simulink library "WECSim_Lib"  (R2019b)
settings: Solver=ode45  StartTime=0.0  StopTime=10.0  RelTol=1e-3  EnableMultiTasking=on
undefined symbols (not defined in the file): body, constraint, mooring, pto, simu, waves, X, Y, Z
libraries: nesl_utility x168, sm_lib x94, vrlib x12
(part 6 of 6)

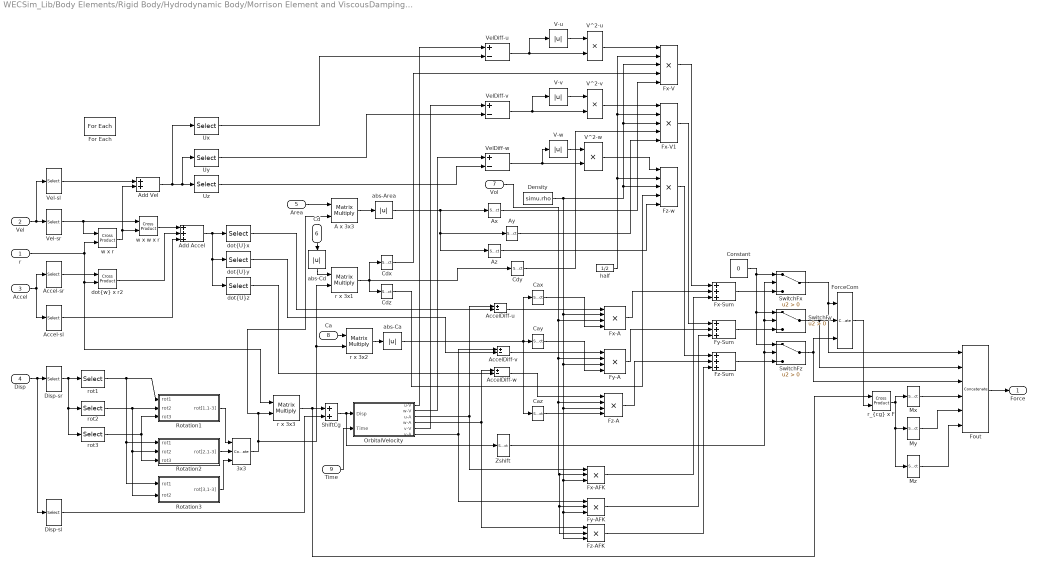
== system WECSim_Lib/Body Elements/Rigid Body/Hydrodynamic Body/Morrison Element and ViscousDampingForceCalculation/Morrison Element Variant Subsystem/Morrison Element On/Regular Wave Morison Force/MorrisonElements ==
  r : Inport  Partition=on  PartitionDimension=1  PartitionWidth=1  PartitionOffset=0
  Vel : Inport  Port=2
  Accel : Inport  Port=3
  Disp : Inport  Port=4
  Area : Inport  Port=5  Partition=on  PartitionDimension=1  PartitionWidth=1  PartitionOffset=0
  Cd : Inport  Port=6  Partition=on  PartitionDimension=1  PartitionWidth=1  PartitionOffset=0
  Vol : Inport  Port=7  Partition=on  PartitionDimension=1  PartitionWidth=1  PartitionOffset=0
  Ca : Inport  Port=8  Partition=on  PartitionDimension=1  PartitionWidth=1  PartitionOffset=0
  Time : Inport  Port=9
  3x3 : Concatenate  NumInputs=3  Mode=Multidimensional array
  A x 3x3 : Product  Multiplication=Matrix(*)
  Accel-sl : Selector  InputPortWidth=6  IndexOptions=Index vector (dialog)  Indices=[1 2 3]  OutputSizes=1
  Accel-sr : Selector  InputPortWidth=6  IndexOptions=Index vector (dialog)  Indices=[4 5 6]  OutputSizes=1
  AccelDiff-u : Sum  Inputs=+-
  AccelDiff-v : Sum  Inputs=+-
  AccelDiff-w : Sum  Inputs=+-
  Add Accel : Sum  Inputs=+++
  Add Vel : Sum
  Ax : Selector  InputPortWidth=3  IndexOptions=Index vector (dialog)  Indices=[1]  OutputSizes=1
  Ay : Selector  InputPortWidth=3  IndexOptions=Index vector (dialog)  Indices=[2]  OutputSizes=1
  Az : Selector  InputPortWidth=3  IndexOptions=Index vector (dialog)  Indices=[3]  OutputSizes=1
  Cax : Selector  InputPortWidth=3  IndexOptions=Index vector (dialog)  Indices=[1]  OutputSizes=1
  Cay : Selector  InputPortWidth=3  IndexOptions=Index vector (dialog)  Indices=[2]  OutputSizes=1
  Caz : Selector  InputPortWidth=3  IndexOptions=Index vector (dialog)  Indices=[3]  OutputSizes=1
  Cdx : Selector  InputPortWidth=3  IndexOptions=Index vector (dialog)  Indices=[1]  OutputSizes=1
  Cdy : Selector  InputPortWidth=3  IndexOptions=Index vector (dialog)  Indices=[2]  OutputSizes=1
  Cdz : Selector  InputPortWidth=3  IndexOptions=Index vector (dialog)  Indices=[3]  OutputSizes=1
  Constant : Constant  Value=0
  Density : Constant  Value=simu.rho
  Disp-sl : Selector  InputPortWidth=6  IndexOptions=Index vector (dialog)  Indices=[1 2 3]  OutputSizes=1
  Disp-sr : Selector  InputPortWidth=6  IndexOptions=Index vector (dialog)  Indices=[4 5 6]  OutputSizes=1
  For Each : ForEach  DisableCoverage=on
  ForceCom : Concatenate  NumInputs=3  ConcatenateDimension=2
  Fout : Concatenate  NumInputs=6  Mode=Multidimensional array  ConcatenateDimension=2
  Fx-A : Product  Inputs=4
  Fx-AFK : Product  Inputs=3
  Fx-Sum : Sum  Inputs=+++
  Fx-V : Product  Inputs=5
  Fx-V1 : Product  Inputs=5
  Fy-A : Product  Inputs=4
  Fy-AFK : Product  Inputs=3
  Fy-Sum : Sum  Inputs=+++
  Fz-A : Product  Inputs=4
  Fz-AFK : Product  Inputs=3
  Fz-Sum : Sum  Inputs=+++
  Fz-w : Product  Inputs=5
  Mx : Selector  InputPortWidth=3  IndexOptions=Index vector (dialog)  Indices=[1]  OutputSizes=1
  My : Selector  InputPortWidth=3  IndexOptions=Index vector (dialog)  Indices=[2]  OutputSizes=1
  Mz : Selector  InputPortWidth=3  IndexOptions=Index vector (dialog)  Indices=[3]  OutputSizes=1
  OrbitalVelocity : Subsystem
  Rotation1 : Subsystem
  Rotation2 : Subsystem
  Rotation3 : Subsystem
  ShiftCg : Sum
  SwitchFx : Switch  Criteria=u2 > Threshold
  SwitchFy : Switch  Criteria=u2 > Threshold
  SwitchFz : Switch  Criteria=u2 > Threshold
  Ux : Selector  InputPortWidth=3  IndexOptions=Index vector (dialog)  Indices=[1]  OutputSizes=1
  Uy : Selector  InputPortWidth=3  IndexOptions=Index vector (dialog)  Indices=[2]  OutputSizes=1
  Uz : Selector  InputPortWidth=3  IndexOptions=Index vector (dialog)  Indices=[3]  OutputSizes=1
  V-u : Abs
  V-v : Abs
  V-w : Abs
  V^2-u : Product
  V^2-v : Product
  V^2-w : Product
  Vel-sl : Selector  InputPortWidth=6  IndexOptions=Index vector (dialog)  Indices=[1 2 3]  OutputSizes=1
  "Vel-sr " : Selector  InputPortWidth=6  IndexOptions=Index vector (dialog)  Indices=[4 5 6]  OutputSizes=1
  VelDiff-u : Sum  Inputs=+-
  VelDiff-v : Sum  Inputs=+-
  VelDiff-w : Sum  Inputs=+-
  Zshift : Selector  InputPortWidth=3  IndexOptions=Index vector (dialog)  Indices=[3]  OutputSizes=1
  abs-Area : Abs
  abs-Ca : Abs
  abs-Cd : Abs
  "dot{U}x" : Selector  InputPortWidth=3  IndexOptions=Index vector (dialog)  Indices=[1]  OutputSizes=1
  "dot{U}y" : Selector  InputPortWidth=3  IndexOptions=Index vector (dialog)  Indices=[2]  OutputSizes=1
  "dot{U}z" : Selector  InputPortWidth=3  IndexOptions=Index vector (dialog)  Indices=[3]  OutputSizes=1
  "dot{w} x r2" : vrlib/Utilities/Cross Product
      settings: SourceProductName=Simulink
  half : Constant  Value=1/2
  r x 3x1 : Product  Multiplication=Matrix(*)
  r x 3x2 : Product  Multiplication=Matrix(*)
  r x 3x3 : Product  Multiplication=Matrix(*)
  "r_{cg} x F" : vrlib/Utilities/Cross Product
      settings: SourceProductName=Simulink
  rot1 : Selector  InputPortWidth=3  IndexOptions=Index vector (dialog)  Indices=[1]  OutputSizes=1
  rot2 : Selector  InputPortWidth=3  IndexOptions=Index vector (dialog)  Indices=[2]  OutputSizes=1
  rot3 : Selector  InputPortWidth=3  IndexOptions=Index vector (dialog)  Indices=[3]  OutputSizes=1
  w x r : vrlib/Utilities/Cross Product
      settings: SourceProductName=Simulink
  w x w x r : vrlib/Utilities/Cross Product
      settings: SourceProductName=Simulink
  Force : Outport  PortDimensions=[1 6]  ConcatenationDimension=1
  wires:
  Vel/1 -> Vel-sl/1, "Vel-sr "/1
  w x r/1 -> Add Vel/2, w x w x r/2
  w x w x r/1 -> Add Accel/1
  "Vel-sr "/1 -> w x w x r/1, w x r/1
  r/1 -> r x 3x3/1, "dot{w} x r2"/2, w x r/2
  Accel/1 -> Accel-sl/1, Accel-sr/1
  Accel-sr/1 -> "dot{w} x r2"/1
  "dot{w} x r2"/1 -> Add Accel/2
  Accel-sl/1 -> Add Accel/3
  Add Accel/1 -> "dot{U}z"/1, "dot{U}y"/1, "dot{U}x"/1
  Vel-sl/1 -> Add Vel/1
  Disp/1 -> Disp-sl/1, Disp-sr/1
  Disp-sr/1 -> rot3/1, rot2/1, rot1/1
  rot3/1 -> Rotation2/3(rot3), Rotation1/3(rot3)
  rot1/1 -> Rotation3/1(rot1), Rotation2/1(rot1), Rotation1/1(rot1)
  rot2/1 -> Rotation3/2(rot2), Rotation2/2(rot2), Rotation1/2(rot2)
  Rotation2/1(rot[2,1-3]) -> 3x3/2
  Rotation1/1(rot[1,1-3]) -> 3x3/1
  Rotation3/1(rot[3,1-3]) -> 3x3/3
  r x 3x3/1 -> "r_{cg} x F"/1, ShiftCg/1
  Disp-sl/1 -> ShiftCg/2
  ShiftCg/1 -> Zshift/1, OrbitalVelocity/1(Disp)
  "dot{U}y"/1 -> AccelDiff-v/2
  "dot{U}x"/1 -> AccelDiff-u/2
  OrbitalVelocity/3(u-A) -> AccelDiff-u/1, Fx-AFK/1
  "dot{U}z"/1 -> AccelDiff-w/2
  Add Vel/1 -> Uy/1, Uz/1, Ux/1
  Uy/1 -> VelDiff-v/2
  Ux/1 -> VelDiff-u/2
  Uz/1 -> VelDiff-w/2
  OrbitalVelocity/1(u-V) -> VelDiff-u/1
  OrbitalVelocity/2(w-V) -> VelDiff-w/1
  VelDiff-w/1 -> V-w/1, V^2-w/2
  V^2-u/1 -> Fx-V/1
  half/1 -> Fz-w/2, Fx-V1/2, Fx-V/2
  Density/1 -> Fy-A/3, Fy-AFK/3, Fz-AFK/3, Fx-AFK/3, Fz-A/3, Fx-A/2, Fz-w/3, Fx-V1/3, Fx-V/3
  V^2-w/1 -> Fz-w/1
  AccelDiff-u/1 -> Fx-A/1
  Vol/1 -> Fy-A/2, Fy-AFK/2, Fz-AFK/2, Fx-AFK/2, Fz-A/2, Fx-A/3
  AccelDiff-w/1 -> Fz-A/1
  OrbitalVelocity/4(w-A) -> Fz-AFK/1, AccelDiff-w/1
  Fx-V/1 -> Fx-Sum/1
  Fx-A/1 -> Fx-Sum/2
  Fx-AFK/1 -> Fx-Sum/3
  Fz-w/1 -> Fz-Sum/1
  Fz-A/1 -> Fz-Sum/2
  Fz-AFK/1 -> Fz-Sum/3
  "r_{cg} x F"/1 -> Mz/1, My/1, Mx/1
  Mx/1 -> Fout/4
  My/1 -> Fout/5
  Mz/1 -> Fout/6
  3x3/1 -> A x 3x3/2, r x 3x3/2, r x 3x2/2, r x 3x1/2
  V-u/1 -> V^2-u/1
  VelDiff-u/1 -> V-u/1, V^2-u/2
  Zshift/1 -> SwitchFy/2, SwitchFx/2, SwitchFz/2
  SwitchFz/1 -> ForceCom/3, Fout/3
  SwitchFx/1 -> Fout/1, ForceCom/1
  Fx-Sum/1 -> SwitchFx/3
  Fz-Sum/1 -> SwitchFz/3
  Az/1 -> Fz-w/5
  Area/1 -> A x 3x3/1
  Ax/1 -> Fx-V/5
  Cdx/1 -> Fx-V/4
  Cdz/1 -> Fz-w/4
  A x 3x3/1 -> abs-Area/1
  abs-Area/1 -> Ay/1, Az/1, Ax/1
  ForceCom/1 -> "r_{cg} x F"/2
  Fout/1 -> Force/1
  Caz/1 -> Fz-A/4
  Cax/1 -> Fx-A/4
  Cd/1 -> abs-Cd/1
  r x 3x1/1 -> Cdy/1, Cdz/1, Cdx/1
  Ca/1 -> r x 3x2/1
  r x 3x2/1 -> abs-Ca/1
  OrbitalVelocity/6(v-A) -> AccelDiff-v/1, Fy-AFK/1
  V^2-v/1 -> Fx-V1/1
  V-v/1 -> V^2-v/1
  VelDiff-v/1 -> V-v/1, V^2-v/2
  OrbitalVelocity/5(v-V) -> VelDiff-v/1
  Ay/1 -> Fx-V1/5
  Cdy/1 -> Fx-V1/4
  SwitchFy/1 -> Fout/2, ForceCom/2
  Fy-Sum/1 -> SwitchFy/3
  Fy-AFK/1 -> Fy-Sum/3
  AccelDiff-v/1 -> Fy-A/1
  Cay/1 -> Fy-A/4
  Fy-A/1 -> Fy-Sum/2
  Fx-V1/1 -> Fy-Sum/1
  Constant/1 -> SwitchFy/1, SwitchFz/1, SwitchFx/1
  V-w/1 -> V^2-w/1
  abs-Ca/1 -> Cax/1, Cay/1, Caz/1
  abs-Cd/1 -> r x 3x1/1
  Time/1 -> OrbitalVelocity/2(Time)

== system WECSim_Lib/Body Elements/Rigid Body/Hydrodynamic Body/Morrison Element and ViscousDampingForceCalculation/Morrison Element Variant Subsystem/Morrison Element On/Irregular Wave Morison Force/MorrisonElements/MorisonElementIrregular ==
  Disp : Inport
  waves.kirr : Inport  Port=2  Partition=on  PartitionDimension=1  PartitionWidth=1  PartitionOffset=0
  waves.w : Inport  Port=3  Partition=on  PartitionDimension=1  PartitionWidth=1  PartitionOffset=0
  waves.A : Inport  Port=4  Partition=on  PartitionDimension=1  PartitionWidth=1  PartitionOffset=0
  waves.Phase : Inport  Port=5  Partition=on  PartitionDimension=1  PartitionWidth=1  PartitionOffset=0
  Time : Inport  Port=6
  For Each : ForEach  DisableCoverage=on
  MATLAB Function : MATLAB Function  TreatAsAtomicUnit=on
  gravity : Constant  Value=simu.g  VectorParams1D=off
  rampTime : Constant  Value=simu.rampTime  VectorParams1D=off
  waterDepth : Constant  Value=waves.waterDepth  VectorParams1D=off
  waveDirection : Constant  Value=waves.waveDir  VectorParams1D=off
  u-V : Outport  ConcatenationDimension=1
  w-V : Outport  Port=2  ConcatenationDimension=1
  x-A : Outport  Port=3  ConcatenationDimension=1
  w-A : Outport  Port=4  ConcatenationDimension=1
  v-V : Outport  Port=5  ConcatenationDimension=1
  y-A : Outport  Port=6  ConcatenationDimension=1
  wires:
  gravity/1 -> MATLAB Function/10(g)
  waterDepth/1 -> MATLAB Function/9(waterDepth)
  waveDirection/1 -> MATLAB Function/8(waveDir)
  rampTime/1 -> MATLAB Function/7(rampT)
  Disp/1 -> MATLAB Function/1(disp)
  waves.w/1 -> MATLAB Function/3(waveFreq)
  waves.A/1 -> MATLAB Function/4(waveAmp)
  waves.Phase/1 -> MATLAB Function/5(phase)
  MATLAB Function/1(u) -> u-V/1
  waves.kirr/1 -> MATLAB Function/2(waveNumber)
  Time/1 -> MATLAB Function/6(time)
  MATLAB Function/2(v) -> v-V/1
  MATLAB Function/5(ya) -> y-A/1
  MATLAB Function/6(za) -> w-A/1
  MATLAB Function/4(xa) -> x-A/1
  MATLAB Function/3(w) -> w-V/1

== system WECSim_Lib/Body Elements/Rigid Body/Hydrodynamic Body/Morrison Element and ViscousDampingForceCalculation/Morrison Element Variant Subsystem/Morrison Element On/Irregular Wave Morison Force/MorrisonElements/Rotation1 ==
  rot1 : Inport
  rot2 : Inport  Port=2
  rot3 : Inport  Port=3
  2 : Product
  3 : Product  Inputs=3
  7 : Product
  8 : Product  Inputs=3
  Combine : Concatenate  NumInputs=3  Mode=Multidimensional array  ConcatenateDimension=2
  Trigonometric Function{,1..2,6,9,11} (6 alike) : Trigonometry  Operator=cos
  Trigonometric Function{3..5,7..8,10} (6 alike) : Trigonometry
  rot11 : Product
  rot12 : Sum
  rot13 : Sum  Inputs=+-
  rot[1,1-3] : Outport
  wires:
  Trigonometric Function/1 -> rot11/1
  Trigonometric Function1/1 -> rot11/2
  rot11/1 -> Combine/1
  Trigonometric Function2/1 -> 2/1
  Trigonometric Function3/1 -> 2/2
  Trigonometric Function4/1 -> 3/1
  Trigonometric Function5/1 -> 3/2
  Trigonometric Function6/1 -> 3/3
  2/1 -> rot12/1
  3/1 -> rot12/2
  rot12/1 -> Combine/2
  Combine/1 -> rot[1,1-3]/1
  rot2/1 -> Trigonometric Function/1, Trigonometric Function5/1, Trigonometric Function10/1
  rot3/1 -> Trigonometric Function1/1, Trigonometric Function3/1, Trigonometric Function6/1, Trigonometric Function11/1, Trigonometric Function8/1
  rot1/1 -> Trigonometric Function2/1, Trigonometric Function4/1, Trigonometric Function9/1, Trigonometric Function7/1
  Trigonometric Function7/1 -> 7/1
  Trigonometric Function8/1 -> 7/2
  Trigonometric Function9/1 -> 8/1
  Trigonometric Function10/1 -> 8/2
  Trigonometric Function11/1 -> 8/3
  7/1 -> rot13/1
  8/1 -> rot13/2
  rot13/1 -> Combine/3

== system WECSim_Lib/Body Elements/Rigid Body/Hydrodynamic Body/Morrison Element and ViscousDampingForceCalculation/Morrison Element Variant Subsystem/Morrison Element On/Irregular Wave Morison Force/MorrisonElements/Rotation2 ==
  rot1 : Inport
  rot2 : Inport  Port=2
  rot3 : Inport  Port=3
  2 : Product
  3 : Product  Inputs=3
  7 : Product
  8 : Product  Inputs=3
  Combine : Concatenate  NumInputs=3  Mode=Multidimensional array  ConcatenateDimension=2
  Gain : Gain  Gain=-1
  Trigonometric Function{,2..3,8..9} (5 alike) : Trigonometry  Operator=cos
  Trigonometric Function{1,4..7,10..11} (7 alike) : Trigonometry
  rot11 : Product
  rot12 : Sum  Inputs=+-
  rot13 : Sum
  rot[2,1-3] : Outport
  wires:
  Trigonometric Function/1 -> Gain/1
  Trigonometric Function1/1 -> rot11/2
  rot11/1 -> Combine/1
  Trigonometric Function2/1 -> 2/1
  Trigonometric Function3/1 -> 2/2
  Trigonometric Function4/1 -> 3/1
  Trigonometric Function5/1 -> 3/2
  Trigonometric Function6/1 -> 3/3
  2/1 -> rot12/1
  3/1 -> rot12/2
  rot12/1 -> Combine/2
  Combine/1 -> rot[2,1-3]/1
  rot2/1 -> Trigonometric Function/1, Trigonometric Function5/1, Trigonometric Function10/1
  rot3/1 -> Trigonometric Function1/1, Trigonometric Function3/1, Trigonometric Function6/1, Trigonometric Function11/1, Trigonometric Function8/1
  rot1/1 -> Trigonometric Function2/1, Trigonometric Function4/1, Trigonometric Function9/1, Trigonometric Function7/1
  Trigonometric Function7/1 -> 7/1
  Trigonometric Function8/1 -> 7/2
  Trigonometric Function9/1 -> 8/1
  Trigonometric Function10/1 -> 8/2
  Trigonometric Function11/1 -> 8/3
  7/1 -> rot13/1
  8/1 -> rot13/2
  rot13/1 -> Combine/3
  Gain/1 -> rot11/1

== system WECSim_Lib/Body Elements/Rigid Body/Hydrodynamic Body/Morrison Element and ViscousDampingForceCalculation/Morrison Element Variant Subsystem/Morrison Element On/Irregular Wave Morison Force/MorrisonElements/Rotation3 ==
  rot1 : Inport
  rot2 : Inport  Port=2
  2 : Product
  7 : Product
  Combine : Concatenate  NumInputs=3  Mode=Multidimensional array  ConcatenateDimension=2
  Gain1 : Gain  Gain=-1
  TrigFun1 : Trigonometry
  TrigFun2 : Trigonometry
  TrigFun3 : Trigonometry  Operator=cos
  TrigFun4 : Trigonometry  Operator=cos
  TrigFun5 : Trigonometry  Operator=cos
  rot[3,1-3] : Outport
  wires:
  TrigFun1/1 -> Combine/1
  TrigFun3/1 -> 2/2
  2/1 -> Combine/2
  Combine/1 -> rot[3,1-3]/1
  rot2/1 -> TrigFun5/1, TrigFun3/1, TrigFun1/1
  TrigFun4/1 -> 7/1
  TrigFun5/1 -> 7/2
  rot1/1 -> TrigFun2/1, TrigFun4/1
  7/1 -> Combine/3
  TrigFun2/1 -> Gain1/1
  Gain1/1 -> 2/1

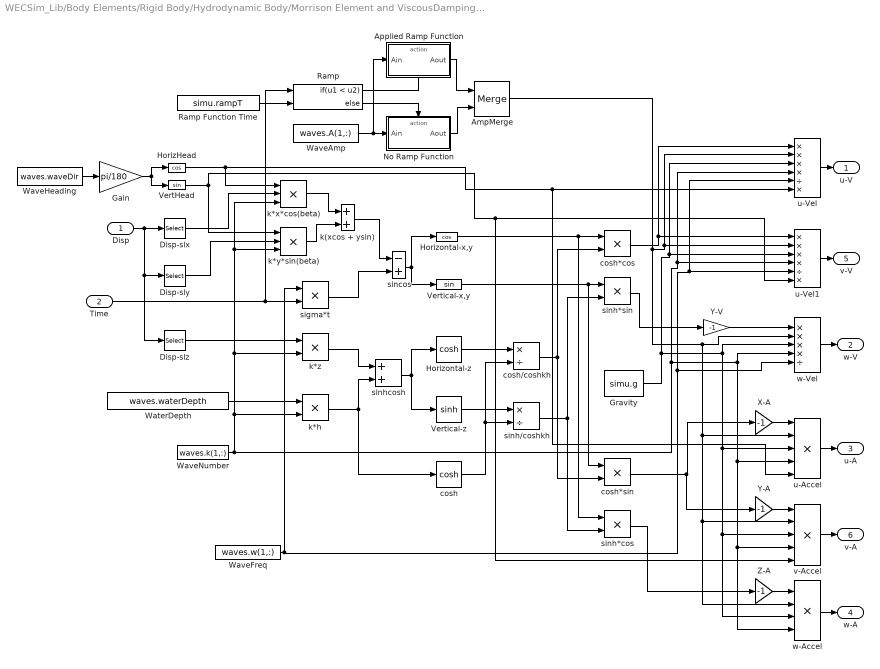
== system WECSim_Lib/Body Elements/Rigid Body/Hydrodynamic Body/Morrison Element and ViscousDampingForceCalculation/Morrison Element Variant Subsystem/Morrison Element On/No Wave Morison Force/MorrisonElements/OrbitalVelocity ==
  Disp : Inport
  Time : Inport  Port=2
  AmpMerge : Merge
  Applied Ramp Function : Subsystem  TreatAsAtomicUnit=on
  Disp-slx : Selector  InputPortWidth=3  IndexOptions=Index vector (dialog)  Indices=[1]  OutputSizes=1
  Disp-sly : Selector  InputPortWidth=3  IndexOptions=Index vector (dialog)  Indices=[2]  OutputSizes=1
  Disp-slz : Selector  InputPortWidth=3  IndexOptions=Index vector (dialog)  Indices=[3]  OutputSizes=1
  Gain : Gain  Gain=pi/180
  Gravity : Constant  Value=simu.g
  HorizHead : Trigonometry  Operator=cos
  Horizontal-x,y : Trigonometry  Operator=cos
  Horizontal-z : Trigonometry  Operator=cosh
  No Ramp Function : Subsystem  TreatAsAtomicUnit=on
  Ramp : If  NumInputs=2  IfExpression=u1 < u2
  Ramp Function Time : Constant  Value=simu.rampT
  VertHead : Trigonometry
  Vertical-x,y : Trigonometry
  Vertical-z : Trigonometry  Operator=sinh
  WaterDepth : Constant  Value=waves.waterDepth
  WaveAmp : Constant  Value=waves.A(1,:)
  WaveFreq : Constant  Value=waves.w(1,:)
  WaveHeading : Constant  Value=waves.waveDir
  WaveNumber : Constant  Value=waves.k(1,:)
  X-A : Gain  Gain=-1
  Y-A : Gain  Gain=-1
  Y-V : Gain  Gain=-1
  Z-A : Gain  Gain=-1
  cosh : Trigonometry  Operator=cosh
  cosh*cos : Product  Inputs=**
  cosh*sin : Product  Inputs=**
  cosh/coshkh : Product  Inputs=*/
  k(xcos + ysin) : Sum
  k*h : Product
  k*x*cos(beta) : Product  Inputs=3
  k*y*sin(beta) : Product  Inputs=3
  k*z : Product
  sigma*t : Product
  sincos : Sum  Inputs=-+
  sinh*cos : Product  Inputs=**
  sinh*sin : Product  Inputs=**
  sinh/coshkh : Product  Inputs=*/
  sinhcosh : Sum
  u-Accel : Product  Inputs=*****
  u-Vel : Product  Inputs=****/*
  u-Vel1 : Product  Inputs=****/*
  v-Accel : Product  Inputs=*****
  w-Accel : Product  Inputs=****
  w-Vel : Product  Inputs=****/
  u-V : Outport
  w-V : Outport  Port=2
  u-A : Outport  Port=3
  w-A : Outport  Port=4
  v-V : Outport  Port=5
  v-A : Outport  Port=6
  wires:
  Disp/1 -> Disp-slz/1, Disp-sly/1, Disp-slx/1
  WaveNumber/1 -> k*h/2, k*z/2, k*y*sin(beta)/3, k*x*cos(beta)/3, w-Vel/4, v-Accel/4, w-Accel/4, u-Accel/4, u-Vel1/4, u-Vel/4
  WaterDepth/1 -> k*h/1
  sigma*t/1 -> sincos/2
  sincos/1 -> Vertical-x,y/1, Horizontal-x,y/1
  k*z/1 -> sinhcosh/1
  k*h/1 -> cosh/1, sinhcosh/2
  sinhcosh/1 -> Vertical-z/1, Horizontal-z/1
  Horizontal-z/1 -> cosh/coshkh/1
  cosh/1 -> sinh/coshkh/2, cosh/coshkh/2
  Vertical-z/1 -> sinh/coshkh/1
  Vertical-x,y/1 -> cosh*sin/1, sinh*sin/1
  sinh/coshkh/1 -> sinh*cos/2, sinh*sin/2
  Horizontal-x,y/1 -> sinh*cos/1, cosh*cos/1
  cosh/coshkh/1 -> cosh*cos/2, cosh*sin/2
  Disp-sly/1 -> k*y*sin(beta)/2
  cosh*cos/1 -> u-Vel1/1, u-Vel/1
  AmpMerge/1 -> w-Vel/2, w-Accel/2, v-Accel/2, u-Accel/2, u-Vel1/2, u-Vel/2
  Gravity/1 -> w-Vel/3, v-Accel/3, w-Accel/3, u-Accel/3, u-Vel1/3, u-Vel/3
  sinh*sin/1 -> Y-V/1
  Y-V/1 -> w-Vel/1
  X-A/1 -> u-Accel/1
  Z-A/1 -> w-Accel/1
  w-Vel/1 -> w-V/1
  u-Accel/1 -> u-A/1
  w-Accel/1 -> w-A/1
  cosh*sin/1 -> Y-A/1, X-A/1
  sinh*cos/1 -> Z-A/1
  Ramp Function Time/1 -> Ramp/2
  Ramp/2 -> No Ramp Function/Action
  Ramp/1 -> Applied Ramp Function/Action
  Time/1 -> Ramp/1, sigma*t/2
  No Ramp Function/1(Aout) -> AmpMerge/2
  Applied Ramp Function/1(Aout) -> AmpMerge/1
  Disp-slz/1 -> k*z/1
  WaveFreq/1 -> w-Vel/5, u-Vel1/5, u-Vel/5, sigma*t/1
  WaveAmp/1 -> Applied Ramp Function/1(Ain), No Ramp Function/1(Ain)
  WaveHeading/1 -> Gain/1
  Gain/1 -> HorizHead/1, VertHead/1
  Disp-slx/1 -> k*x*cos(beta)/2
  HorizHead/1 -> u-Accel/5, u-Vel/6, k*x*cos(beta)/1
  VertHead/1 -> k*y*sin(beta)/1, u-Vel1/6, v-Accel/5
  k*y*sin(beta)/1 -> k(xcos + ysin)/2
  k*x*cos(beta)/1 -> k(xcos + ysin)/1
  k(xcos + ysin)/1 -> sincos/1
  u-Vel1/1 -> v-V/1
  u-Vel/1 -> u-V/1
  Y-A/1 -> v-Accel/1
  v-Accel/1 -> v-A/1

== system WECSim_Lib/Body Elements/Rigid Body/Hydrodynamic Body/Morrison Element and ViscousDampingForceCalculation/Morrison Element Variant Subsystem/Morrison Element On/No Wave Morison Force/MorrisonElements/Rotation1 ==
  rot1 : Inport
  rot2 : Inport  Port=2
  rot3 : Inport  Port=3
  2 : Product
  3 : Product  Inputs=3
  7 : Product
  8 : Product  Inputs=3
  Combine : Concatenate  NumInputs=3  Mode=Multidimensional array  ConcatenateDimension=2
  Trigonometric Function{,1..2,6,9,11} (6 alike) : Trigonometry  Operator=cos
  Trigonometric Function{3..5,7..8,10} (6 alike) : Trigonometry
  rot11 : Product
  rot12 : Sum
  rot13 : Sum  Inputs=+-
  rot[1,1-3] : Outport
  wires:
  Trigonometric Function/1 -> rot11/1
  Trigonometric Function1/1 -> rot11/2
  rot11/1 -> Combine/1
  Trigonometric Function2/1 -> 2/1
  Trigonometric Function3/1 -> 2/2
  Trigonometric Function4/1 -> 3/1
  Trigonometric Function5/1 -> 3/2
  Trigonometric Function6/1 -> 3/3
  2/1 -> rot12/1
  3/1 -> rot12/2
  rot12/1 -> Combine/2
  Combine/1 -> rot[1,1-3]/1
  rot2/1 -> Trigonometric Function/1, Trigonometric Function5/1, Trigonometric Function10/1
  rot3/1 -> Trigonometric Function1/1, Trigonometric Function3/1, Trigonometric Function6/1, Trigonometric Function11/1, Trigonometric Function8/1
  rot1/1 -> Trigonometric Function2/1, Trigonometric Function4/1, Trigonometric Function9/1, Trigonometric Function7/1
  Trigonometric Function7/1 -> 7/1
  Trigonometric Function8/1 -> 7/2
  Trigonometric Function9/1 -> 8/1
  Trigonometric Function10/1 -> 8/2
  Trigonometric Function11/1 -> 8/3
  7/1 -> rot13/1
  8/1 -> rot13/2
  rot13/1 -> Combine/3

== system WECSim_Lib/Body Elements/Rigid Body/Hydrodynamic Body/Morrison Element and ViscousDampingForceCalculation/Morrison Element Variant Subsystem/Morrison Element On/No Wave Morison Force/MorrisonElements/Rotation2 ==
  rot1 : Inport
  rot2 : Inport  Port=2
  rot3 : Inport  Port=3
  2 : Product
  3 : Product  Inputs=3
  7 : Product
  8 : Product  Inputs=3
  Combine : Concatenate  NumInputs=3  Mode=Multidimensional array  ConcatenateDimension=2
  Gain : Gain  Gain=-1
  Trigonometric Function{,2..3,8..9} (5 alike) : Trigonometry  Operator=cos
  Trigonometric Function{1,4..7,10..11} (7 alike) : Trigonometry
  rot11 : Product
  rot12 : Sum  Inputs=+-
  rot13 : Sum
  rot[2,1-3] : Outport
  wires:
  Trigonometric Function/1 -> Gain/1
  Trigonometric Function1/1 -> rot11/2
  rot11/1 -> Combine/1
  Trigonometric Function2/1 -> 2/1
  Trigonometric Function3/1 -> 2/2
  Trigonometric Function4/1 -> 3/1
  Trigonometric Function5/1 -> 3/2
  Trigonometric Function6/1 -> 3/3
  2/1 -> rot12/1
  3/1 -> rot12/2
  rot12/1 -> Combine/2
  Combine/1 -> rot[2,1-3]/1
  rot2/1 -> Trigonometric Function/1, Trigonometric Function5/1, Trigonometric Function10/1
  rot3/1 -> Trigonometric Function1/1, Trigonometric Function3/1, Trigonometric Function6/1, Trigonometric Function11/1, Trigonometric Function8/1
  rot1/1 -> Trigonometric Function2/1, Trigonometric Function4/1, Trigonometric Function9/1, Trigonometric Function7/1
  Trigonometric Function7/1 -> 7/1
  Trigonometric Function8/1 -> 7/2
  Trigonometric Function9/1 -> 8/1
  Trigonometric Function10/1 -> 8/2
  Trigonometric Function11/1 -> 8/3
  7/1 -> rot13/1
  8/1 -> rot13/2
  rot13/1 -> Combine/3
  Gain/1 -> rot11/1

== system WECSim_Lib/Body Elements/Rigid Body/Hydrodynamic Body/Morrison Element and ViscousDampingForceCalculation/Morrison Element Variant Subsystem/Morrison Element On/No Wave Morison Force/MorrisonElements/Rotation3 ==
  rot1 : Inport
  rot2 : Inport  Port=2
  2 : Product
  7 : Product
  Combine : Concatenate  NumInputs=3  Mode=Multidimensional array  ConcatenateDimension=2
  Gain1 : Gain  Gain=-1
  TrigFun1 : Trigonometry
  TrigFun2 : Trigonometry
  TrigFun3 : Trigonometry  Operator=cos
  TrigFun4 : Trigonometry  Operator=cos
  TrigFun5 : Trigonometry  Operator=cos
  rot[3,1-3] : Outport
  wires:
  TrigFun1/1 -> Combine/1
  TrigFun3/1 -> 2/2
  2/1 -> Combine/2
  Combine/1 -> rot[3,1-3]/1
  rot2/1 -> TrigFun5/1, TrigFun3/1, TrigFun1/1
  TrigFun4/1 -> 7/1
  TrigFun5/1 -> 7/2
  rot1/1 -> TrigFun2/1, TrigFun4/1
  7/1 -> Combine/3
  TrigFun2/1 -> Gain1/1
  Gain1/1 -> 2/1

== system WECSim_Lib/Body Elements/Rigid Body/Hydrodynamic Body/Morrison Element and ViscousDampingForceCalculation/Morrison Element Variant Subsystem/Morrison Element On/Regular Wave Morison Force/MorrisonElements/OrbitalVelocity ==
  Disp : Inport
  Time : Inport  Port=2
  MATLAB Function : MATLAB Function  TreatAsAtomicUnit=on
  WaveAmp : Constant  Value=waves.A(1,:)
  WaveFreq : Constant  Value=waves.w(1,:)
  WaveNumber : Constant  Value=waves.k(1,:)
  gravity : Constant  Value=simu.g  VectorParams1D=off
  phase : Constant  Value=0
  rampTime : Constant  Value=simu.rampTime  VectorParams1D=off
  waterDepth : Constant  Value=waves.waterDepth  VectorParams1D=off
  waveDirection : Constant  Value=waves.waveDir  VectorParams1D=off
  u-V : Outport
  w-V : Outport  Port=2
  u-A : Outport  Port=3
  w-A : Outport  Port=4
  v-V : Outport  Port=5
  v-A : Outport  Port=6
  wires:
  Disp/1 -> MATLAB Function/1(disp)
  phase/1 -> MATLAB Function/5(randPhase)
  WaveNumber/1 -> MATLAB Function/2(waveNumber)
  WaveFreq/1 -> MATLAB Function/3(waveFreq)
  WaveAmp/1 -> MATLAB Function/4(waveAmp)
  Time/1 -> MATLAB Function/6(time)
  gravity/1 -> MATLAB Function/10(g)
  waterDepth/1 -> MATLAB Function/9(waterDepth)
  waveDirection/1 -> MATLAB Function/8(waveDir)
  rampTime/1 -> MATLAB Function/7(rampT)
  MATLAB Function/3(w) -> w-V/1
  MATLAB Function/4(xa) -> u-A/1
  MATLAB Function/6(za) -> w-A/1
  MATLAB Function/2(v) -> v-V/1
  MATLAB Function/1(u) -> u-V/1
  MATLAB Function/5(ya) -> v-A/1

== system WECSim_Lib/Body Elements/Rigid Body/Hydrodynamic Body/Morrison Element and ViscousDampingForceCalculation/Morrison Element Variant Subsystem/Morrison Element On/Regular Wave Morison Force/MorrisonElements/Rotation1 ==
  rot1 : Inport
  rot2 : Inport  Port=2
  rot3 : Inport  Port=3
  2 : Product
  3 : Product  Inputs=3
  7 : Product
  8 : Product  Inputs=3
  Combine : Concatenate  NumInputs=3  Mode=Multidimensional array  ConcatenateDimension=2
  Trigonometric Function{,1..2,6,9,11} (6 alike) : Trigonometry  Operator=cos
  Trigonometric Function{3..5,7..8,10} (6 alike) : Trigonometry
  rot11 : Product
  rot12 : Sum
  rot13 : Sum  Inputs=+-
  rot[1,1-3] : Outport
  wires:
  Trigonometric Function/1 -> rot11/1
  Trigonometric Function1/1 -> rot11/2
  rot11/1 -> Combine/1
  Trigonometric Function2/1 -> 2/1
  Trigonometric Function3/1 -> 2/2
  Trigonometric Function4/1 -> 3/1
  Trigonometric Function5/1 -> 3/2
  Trigonometric Function6/1 -> 3/3
  2/1 -> rot12/1
  3/1 -> rot12/2
  rot12/1 -> Combine/2
  Combine/1 -> rot[1,1-3]/1
  rot2/1 -> Trigonometric Function/1, Trigonometric Function5/1, Trigonometric Function10/1
  rot3/1 -> Trigonometric Function1/1, Trigonometric Function3/1, Trigonometric Function6/1, Trigonometric Function11/1, Trigonometric Function8/1
  rot1/1 -> Trigonometric Function2/1, Trigonometric Function4/1, Trigonometric Function9/1, Trigonometric Function7/1
  Trigonometric Function7/1 -> 7/1
  Trigonometric Function8/1 -> 7/2
  Trigonometric Function9/1 -> 8/1
  Trigonometric Function10/1 -> 8/2
  Trigonometric Function11/1 -> 8/3
  7/1 -> rot13/1
  8/1 -> rot13/2
  rot13/1 -> Combine/3

== system WECSim_Lib/Body Elements/Rigid Body/Hydrodynamic Body/Morrison Element and ViscousDampingForceCalculation/Morrison Element Variant Subsystem/Morrison Element On/Regular Wave Morison Force/MorrisonElements/Rotation2 ==
  rot1 : Inport
  rot2 : Inport  Port=2
  rot3 : Inport  Port=3
  2 : Product
  3 : Product  Inputs=3
  7 : Product
  8 : Product  Inputs=3
  Combine : Concatenate  NumInputs=3  Mode=Multidimensional array  ConcatenateDimension=2
  Gain : Gain  Gain=-1
  Trigonometric Function{,2..3,8..9} (5 alike) : Trigonometry  Operator=cos
  Trigonometric Function{1,4..7,10..11} (7 alike) : Trigonometry
  rot11 : Product
  rot12 : Sum  Inputs=+-
  rot13 : Sum
  rot[2,1-3] : Outport
  wires:
  Trigonometric Function/1 -> Gain/1
  Trigonometric Function1/1 -> rot11/2
  rot11/1 -> Combine/1
  Trigonometric Function2/1 -> 2/1
  Trigonometric Function3/1 -> 2/2
  Trigonometric Function4/1 -> 3/1
  Trigonometric Function5/1 -> 3/2
  Trigonometric Function6/1 -> 3/3
  2/1 -> rot12/1
  3/1 -> rot12/2
  rot12/1 -> Combine/2
  Combine/1 -> rot[2,1-3]/1
  rot2/1 -> Trigonometric Function/1, Trigonometric Function5/1, Trigonometric Function10/1
  rot3/1 -> Trigonometric Function1/1, Trigonometric Function3/1, Trigonometric Function6/1, Trigonometric Function11/1, Trigonometric Function8/1
  rot1/1 -> Trigonometric Function2/1, Trigonometric Function4/1, Trigonometric Function9/1, Trigonometric Function7/1
  Trigonometric Function7/1 -> 7/1
  Trigonometric Function8/1 -> 7/2
  Trigonometric Function9/1 -> 8/1
  Trigonometric Function10/1 -> 8/2
  Trigonometric Function11/1 -> 8/3
  7/1 -> rot13/1
  8/1 -> rot13/2
  rot13/1 -> Combine/3
  Gain/1 -> rot11/1

== system WECSim_Lib/Body Elements/Rigid Body/Hydrodynamic Body/Morrison Element and ViscousDampingForceCalculation/Morrison Element Variant Subsystem/Morrison Element On/Regular Wave Morison Force/MorrisonElements/Rotation3 ==
  rot1 : Inport
  rot2 : Inport  Port=2
  2 : Product
  7 : Product
  Combine : Concatenate  NumInputs=3  Mode=Multidimensional array  ConcatenateDimension=2
  Gain1 : Gain  Gain=-1
  TrigFun1 : Trigonometry
  TrigFun2 : Trigonometry
  TrigFun3 : Trigonometry  Operator=cos
  TrigFun4 : Trigonometry  Operator=cos
  TrigFun5 : Trigonometry  Operator=cos
  rot[3,1-3] : Outport
  wires:
  TrigFun1/1 -> Combine/1
  TrigFun3/1 -> 2/2
  2/1 -> Combine/2
  Combine/1 -> rot[3,1-3]/1
  rot2/1 -> TrigFun5/1, TrigFun3/1, TrigFun1/1
  TrigFun4/1 -> 7/1
  TrigFun5/1 -> 7/2
  rot1/1 -> TrigFun2/1, TrigFun4/1
  7/1 -> Combine/3
  TrigFun2/1 -> Gain1/1
  Gain1/1 -> 2/1

== system WECSim_Lib/Body Elements/Rigid Body/Hydrodynamic Body/Morrison Element and ViscousDampingForceCalculation/Morrison Element Variant Subsystem/Morrison Element On/No Wave Morison Force/MorrisonElements/OrbitalVelocity/Applied Ramp Function ==
  Ain : Inport
  Action Port : ActionPort
  Add : Sum
  Constant : Constant  Value=2
  Constant1 : Constant
  Divide : Product  Inputs=**/
  Sine Wave : Sin  Frequency=pi/simu.rampT  Phase=pi+pi/2  SampleTime=0
  Aout : Outport
  wires:
  Ain/1 -> Divide/1
  Divide/1 -> Aout/1
  Constant/1 -> Divide/3
  Constant1/1 -> Add/1
  Sine Wave/1 -> Add/2
  Add/1 -> Divide/2

== system WECSim_Lib/Body Elements/Rigid Body/Hydrodynamic Body/Morrison Element and ViscousDampingForceCalculation/Morrison Element Variant Subsystem/Morrison Element On/No Wave Morison Force/MorrisonElements/OrbitalVelocity/No Ramp Function ==
  Ain : Inport
  Action Port : ActionPort
  Aout : Outport
  wires:
  Ain/1 -> Aout/1

== matlab function WECSim_Lib/Body Elements/Rigid Body/Hydrodynamic Body/Hydrostatic Restoring Force Calculation/Linear and Nonlinear Restoring Force Variant Subsystem/Nonlinear Hydrostatic Restoring Force/Restoring Forces ==
  data: x input; elv input; center input; f output; tnorm input; area input; rho input; g input; cg input; p output; mass input
function [f,p]  = nonLinearBuoyancy(x,elv,center,tnorm,area,rho,g,cg,mass)
% Function to calculate buoyancy force and moment on a triangulated surface
% NOTE: This function assumes that the STL file is imported with its CG at 0,0,0
[f,p] = calc_buoyancy(x,elv,center,tnorm,area,rho,g,cg);
f = -f + [0 0 g*mass 0 0 0]';
end


function [f,p] = calc_buoyancy(x,elv,center,tnorm,area,rho,g,cg)
% Function to apply translation and rotation and calculate forces

% Compute new tri coords after cog rotation and translation
center = rotateXYZ(center,[1 0 0],x(4));
center = rotateXYZ(center,[0 1 0],x(5));
center = rotateXYZ(center,[0 0 1],x(6));
center = offsetXYZ(center,x);
center = offsetXYZ(center,cg);
% Compute new normal vectors coords after cog rotation
tnorm = rotateXYZ(tnorm,[1 0 0],x(4));
tnorm = rotateXYZ(tnorm,[0 1 0],x(5));
tnorm = rotateXYZ(tnorm,[0 0 1],x(6));

% Calculate the hydrostatic forces
av = tnorm .* [area area area];
[f,p]=fHydrostatic(center,elv,x(1:3)+cg,av,rho,g);
end

function verts = offsetXYZ(verts,x)
% Function to move the position vertices
verts(:,1) = verts(:,1) + x(1);
verts(:,2) = verts(:,2) + x(2);
verts(:,3) = verts(:,3) + x(3);
end

function xn = rotateXYZ(x,ax,t)
% Function to rotate a point about an arbitrary axis
% x: 3-componenet coordiantes
% ax: axis about which to rotate (must be a vector length 1)
% t: rotation angle
% xn: new coordinates after rotation
rotMat = zeros(3);
rotMat(1,1) = ax(1)*ax(1)*(1-cos(t))    + cos(t);
rotMat(1,2) = ax(2)*ax(1)*(1-cos(t))    + ax(3)*sin(t);
rotMat(1,3) = ax(3)*ax(1)*(1-cos(t))    - ax(2)*sin(t);
rotMat(2,1) = ax(1)*ax(2)*(1-cos(t))    - ax(3)*sin(t);
rotMat(2,2) = ax(2)*ax(2)*(1-cos(t))    + cos(t);
rotMat(2,3) = ax(3)*ax(2)*(1-cos(t))    + ax(1)*sin(t);
rotMat(3,1) = ax(1)*ax(3)*(1-cos(t))    + ax(2)*sin(t);
rotMat(3,2) = ax(2)*ax(3)*(1-cos(t))    - ax(1)*sin(t);
rotMat(3,3) = ax(3)*ax(3)*(1-cos(t))    + cos(t);
xn = x*rotMat;
end

function [f,p] = fHydrostatic(center,elv,instcg,av,rho,g)
% Function to calculate the force and moment about the cog due to hydrostatic pressure
f = zeros(6,1);

% Zeor out regions above the mean free surface
z=center(:,3); z((z-elv)>0)=0;

% Calculate the hydrostatic pressure at each triangle center
pressureVect = rho*g.*[-z -z -z].*-av;
p = rho*g.*-z;
% Compute force about cog
f(1:3) = sum(pressureVect);

tmp1 = ones(length(center(:,1)),1);
tmp2 = tmp1*instcg';
center2cgVec = center-tmp2;

f(4:6)= sum(cross(center2cgVec,pressureVect));
end

== matlab function WECSim_Lib/Body Elements/Rigid Body/Hydrodynamic Body/Morrison Element and ViscousDampingForceCalculation/Morrison Element Variant Subsystem/Morrison Element On/Irregular Wave Morison Force/MorrisonElements/MorisonElementIrregular/MATLAB Function ==
  data: u output; v output; disp input size=[1 3]; waveNumber input; waveFreq input; waveAmp input; phase input; time input; rampT input size=[1 1]; waveDir input size=[1 1]; waterDepth input size=[1 1]; g input size=[1 1]; w output; xa output; ya output; za output
function [u,v,w,xa,ya,za] = calc_orbital_vel(disp, waveNumber, waveFreq, waveAmp, phase, time, rampT, waveDir, waterDepth, g)
%#codegen

[u,v,w,xa,ya,za] = orbital_velocity(disp, waveNumber, waveFreq, waveAmp, phase, time, rampT, waveDir, waterDepth, g);

== matlab function WECSim_Lib/Body Elements/Rigid Body/Hydrodynamic Body/Wave Radiation Forces Calculation/SS CI and Constant-Damping-CoeVariant Subsystem/Convolution Integral Calculation/MATLAB Function ==
  data: v input double; F_FM output double size=[6 1]; IRKB parameter double; lenJ parameter double size=1; CTTime parameter double
function F_FM = ConvolutionIntegral_interp(v, IRKB, lenJ, CTTime)
%#codegen
% Function to calculate convolution integral

%define persistent variables
interp_factor = 1;
persistent velocity IRKB_interp CTTime_interp;

if isempty(velocity) 
    CTTime_interp  = CTTime(1:interp_factor:end);
    velocity       = zeros(lenJ,length(CTTime_interp));
    IRKB_reordered = permute(IRKB,[3 1 2]);                     % permutes from [601 6 12] to [12 601 6]
    IRKB_interp    = IRKB_reordered(:,1:interp_factor:end, :);  % what does this do?
end 
% shift velocity
velocity      = circshift(velocity, 1, 2);
v = v(:)'';           %force v to be a column
velocity(:,1) = v(:);

%integrate
time_series = bsxfun(@times, IRKB_interp, velocity);
F_FM = squeeze(trapz(CTTime_interp,sum(time_series, 1)));

end

== matlab function WECSim_Lib/Moorings/MoorDyn/Structure/Motion Sensor/Angle ==
  data: Q input; E output
function E  = EulerAngle(Q)
%#codegen
E=zeros(3,1);
E(1) = atan2( (2*(Q(1)*Q(2)+Q(3)*Q(4))), (1-2* (Q(2)^2+Q(3)^2) ) );
E(2) = asin( 2* (Q(1)*Q(3) - Q(4)*Q(2)));
E(3) = atan2( (2*(Q(1)*Q(4)+Q(2)*Q(3))), (1-2* (Q(3)^2+Q(4)^2) ) );

== matlab function WECSim_Lib/Moorings/MoorDyn/MoorDyn/MoorDyn/Triggered Subsystem/MATLAB Function ==
  data: X input; FLines output; XD input; Time input; CoupTime input
function FLines  = MoorDyn_matlab_FCN(X,XD,Time,CoupTime)

    FLines = zeros(1,6);
    coder.extrinsic('MoorDyn_caller');
    
    FLines = MoorDyn_caller(X,XD,Time-CoupTime,CoupTime);

== matlab function WECSim_Lib/Moorings/MooringMatrix/Structure/Motion Sensor/Angle ==
  data: Q input; E output
function E  = EulerAngle(Q)
%#codegen
E=zeros(3,1);
E(1) = atan2( (2*(Q(1)*Q(2)+Q(3)*Q(4))), (1-2* (Q(2)^2+Q(3)^2) ) );
E(2) = asin( 2* (Q(1)*Q(3) - Q(4)*Q(2)));
E(3) = atan2( (2*(Q(1)*Q(4)+Q(2)*Q(3))), (1-2* (Q(3)^2+Q(4)^2) ) );

== matlab function WECSim_Lib/Body Elements/Rigid Body/Hydrodynamic Body/Morrison Element and ViscousDampingForceCalculation/Morrison Element Variant Subsystem/Morrison Element On/Regular Wave Morison Force/MorrisonElements/OrbitalVelocity/MATLAB Function ==
  data: u output; v output; disp input size=[1 3]; waveNumber input size=[1 1]; waveFreq input size=[1 1]; waveAmp input size=[1 1]; randPhase input; time input; rampT input size=[1 1]; waveDir input size=[1 1]; waterDepth input size=[1 1]; g input size=[1 1]; w output; xa output; ya output; za output
function [u,v,w,xa,ya,za] = calc_orbital_vel(disp, waveNumber, waveFreq, waveAmp, randPhase, time, rampT, waveDir, waterDepth, g)
%#codegen

[u,v,w,xa,ya,za] = orbital_velocity(disp, waveNumber, waveFreq, waveAmp, randPhase, time, rampT, waveDir, waterDepth, g);

== matlab function WECSim_Lib/Body Elements/Rigid Body/Hydrodynamic Body/Nonlinear Wave Elevation/Linear or Instantaneous Free Surface/Instantaneous Water Free Surface  /Instantaneous FS ==
  data: x input; center input; f output; cg input; AH input; w input; dw input; k input; typeNum input; t input; rampT input; phaseRand input; waveDir input
function f  = waveElevation(x,center,cg,AH,w,dw,k,typeNum,t,rampT,phaseRand,waveDir)
% Function to calculate the wave elevation at the ceontroids of triangulated surface
% NOTE: This function assumes that the STL file is imported with its CG at 0,0,0
f = calc_elev(x,center,cg,AH,w,dw,k,typeNum,t,rampT,phaseRand, waveDir);
end

function f = calc_elev(x,center,cg,AH,w,dw,k,typeNum,t,rampT,phaseRand,waveDir)
% Function to rotate and translate body and call wave elevation function at new locations

% Compute new tri center coords after cog rotation and translation
center = rotateXYZ(center,[1 0 0],x(4));
center = rotateXYZ(center,[0 1 0],x(5));
center = rotateXYZ(center,[0 0 1],x(6));
center = offsetXYZ(center,x);
center = offsetXYZ(center,cg);
% Calculate the free surface
f=waveElev(center,AH,w,dw,t,k,rampT,phaseRand,typeNum,waveDir);
end

function verts = offsetXYZ(verts,x)
% Function to move the position vertices
verts(:,1) = verts(:,1) + x(1);
verts(:,2) = verts(:,2) + x(2);
verts(:,3) = verts(:,3) + x(3);
end

function xn = rotateXYZ(x,ax,t)
% Function to rotate a point about an arbitrary axis
% x: 3-component coordinates
% ax: axis about which to rotate (must be a vector length 1)
% t: rotation angle
% xn: new coordinates after rotation
rotMat = zeros(3);
rotMat(1,1) = ax(1)*ax(1)*(1-cos(t))    + cos(t);
rotMat(1,2) = ax(2)*ax(1)*(1-cos(t))    + ax(3)*sin(t);
rotMat(1,3) = ax(3)*ax(1)*(1-cos(t))    - ax(2)*sin(t);
rotMat(2,1) = ax(1)*ax(2)*(1-cos(t))    - ax(3)*sin(t);
rotMat(2,2) = ax(2)*ax(2)*(1-cos(t))    + cos(t);
rotMat(2,3) = ax(3)*ax(2)*(1-cos(t))    + ax(1)*sin(t);
rotMat(3,1) = ax(1)*ax(3)*(1-cos(t))    + ax(2)*sin(t);
rotMat(3,2) = ax(2)*ax(3)*(1-cos(t))    - ax(1)*sin(t);
rotMat(3,3) = ax(3)*ax(3)*(1-cos(t))    + cos(t);
xn = x*rotMat;
end

function f=waveElev(center,AH,w,dw,t,k,rampT,phaseRand,typeNum,waveDir)
% Function to calculate the wave elevation at an array of points
f = zeros(length(center(:,3)),1);
cx = center(:,1);
cy = center(:,2);
X = cx*cos(waveDir*pi/180) + cy*sin(waveDir*pi/180);
if typeNum <10
elseif typeNum <20
    f = AH(1).*cos(k(1).*X-w(1)*t);
elseif typeNum <30
    tmp=sqrt(AH.*dw);
    tmp1 = ones(1,length(center(:,1)));
    tmp2 = (w.*t+phaseRand)*tmp1;
    tmp3 = cos(k*X'- tmp2);
    f(:,1) = tmp3'*tmp;
end
if t<=rampT
    rampF = (1+cos(pi+pi*t/rampT))/2;
    f = f.*rampF;
end
end

== matlab function WECSim_Lib/Body Elements/Rigid Body/Hydrodynamic Body/Structure/Motion Sensor/Angle ==
  data: Q input; E output
function E  = EulerAngle(Q)
% Euler Angle Type II or Tait-Bryan Angle for sequence 321 or zyx (Nautical or Cardan angles).
% Yaw [-180,180], followed by pitch [-90,90], followed by roll [-180,180]
E = zeros(3,1);
E(1) = atan2((2*(Q(1)*Q(2)+Q(3)*Q(4))),(1-2*(Q(2)^2+Q(3)^2)));
E(2) = asin(2*(Q(1)*Q(3)-Q(4)*Q(2)));
E(3) = atan2((2*(Q(1)*Q(4)+Q(2)*Q(3))),(1-2*(Q(3)^2+Q(4)^2)));

== matlab function WECSim_Lib/Body Elements/Rigid Body/Hydrodynamic Body/Wave Diffraction and Excitation Force Calculation/Linear Wave Excitation Force Variant Subsystem/Irregular Wave Excitation Force/MATLAB Function ==
  data: A input; Fext output; w input; fExtRE input; fExtIM input; phaseRand input; dw input; time input
function Fext = fcn(A,w,fExtRE,fExtIM,phaseRand,dw,time)
%#codegen

persistent A1 B1 B11 C1 D1 D11 E1 E11

A1=bsxfun(@plus,w*time,pi/2);
B1= sin(bsxfun(@plus,A1,phaseRand));
B11 = sin(bsxfun(@plus,w*time,phaseRand));
C1 = sqrt(bsxfun(@times,A,dw));
D1 =bsxfun(@times,fExtRE,C1);
D11 = bsxfun(@times,fExtIM,C1);
E1 = bsxfun(@times,B1,D1);
E11 = bsxfun(@times,B11,D11);

Fext = sum(bsxfun(@minus,E1,E11));

== matlab function WECSim_Lib/Body Elements/Rigid Body/Hydrodynamic Body/Wave Diffraction and Excitation Force Calculation/Nonlinear FK Force Variant Subsystem/With Nonlinear FroudeKrylov Force/Diffraction and Excitation Forces ==
  data: x input; elv input; center input; f output; tnorm input; area input; rho input; g input; cg input; AH input; w input; dw input; wDepth input; deepWaterWave input; k input; typeNum input; t input; phaseRand input; wp output; wpMeanFS output
function [f, wp, wpMeanFS]  = nonFKForce(x,elv,center,tnorm,area,rho,g,cg,AH,w,dw,wDepth,deepWaterWave,k,typeNum,t,phaseRand)
% Function to calculate wave exitation force and moment on a triangulated surface
% NOTE: This function assumes that the STL file is imported with its CG at 0,0,0

% Logic to calculate nonFKForce at reduced sample time
[f, wp, wpMeanFS] = calc_force(x,elv,center,tnorm,area,rho,g,cg,AH,w,dw,wDepth,deepWaterWave,k,typeNum,t,phaseRand);
end

function [f, wp, wpMeanFS]  = calc_force(x,elv,center,tnorm,area,rho,g,cg,AH,w,dw,wDepth,deepWaterWave,k,typeNum,t,phaseRand)
% Function to apply translation and rotation, and calculate forces.

% Compute new tri coords after cog rotation and translation
centerMeanFS = offsetXYZ(center,cg);
avMeanFS     = tnorm .* [area area area];

% Compute new tri coords after cog rotation and translation
center = rotateXYZ(center,[1 0 0],x(4));
center = rotateXYZ(center,[0 1 0],x(5));
center = rotateXYZ(center,[0 0 1],x(6));
center = offsetXYZ(center,x);
center = offsetXYZ(center,cg);
% Compute new normal vectors coords after cog rotation and translation
tnorm = rotateXYZ(tnorm,[1 0 0],x(4));
tnorm = rotateXYZ(tnorm,[0 1 0],x(5));
tnorm = rotateXYZ(tnorm,[0 0 1],x(6));

% Copute area vectors
av = tnorm .* [area area area];

% Calculate the free surface
wpMeanFS=pDis(centerMeanFS,       0,AH,w,dw,wDepth,deepWaterWave,t,k,phaseRand,typeNum,rho,g);
wp      =pDis(center      ,     elv,AH,w,dw,wDepth,deepWaterWave,t,k,phaseRand,typeNum,rho,g);

% Calculate forces
f_linear   =FK(centerMeanFS,       cg,avMeanFS,wpMeanFS);
f_nonLinear=FK(center      ,x(1:3)+cg,av      ,wp      );
f = f_nonLinear-f_linear;
end

function verts = offsetXYZ(verts,x)
% Function to move the position vertices
verts(:,1) = verts(:,1) + x(1);
verts(:,2) = verts(:,2) + x(2);
verts(:,3) = verts(:,3) + x(3);
end

function xn = rotateXYZ(x,ax,t)
% Function to rotate a point about an arbitrary axis
% x: 3-componenet coordinates
% ax: axis about which to rotate (must be a vector length 1)
% t: rotation angle
% xn: new coordinates after rotation
rotMat = zeros(3);
rotMat(1,1) = ax(1)*ax(1)*(1-cos(t))    + cos(t);
rotMat(1,2) = ax(2)*ax(1)*(1-cos(t))    + ax(3)*sin(t);
rotMat(1,3) = ax(3)*ax(1)*(1-cos(t))    - ax(2)*sin(t);
rotMat(2,1) = ax(1)*ax(2)*(1-cos(t))    - ax(3)*sin(t);
rotMat(2,2) = ax(2)*ax(2)*(1-cos(t))    + cos(t);
rotMat(2,3) = ax(3)*ax(2)*(1-cos(t))    + ax(1)*sin(t);
rotMat(3,1) = ax(1)*ax(3)*(1-cos(t))    + ax(2)*sin(t);
rotMat(3,2) = ax(2)*ax(3)*(1-cos(t))    - ax(1)*sin(t);
rotMat(3,3) = ax(3)*ax(3)*(1-cos(t))    + cos(t);
xn = x*rotMat;
end

function f=pDis(center,elv,AH,w,dw,wDepth,deepWaterWave,t,k,phaseRand,typeNum,rho,g)
% Function to calculate pressure distribution
f = zeros(length(center(:,3)),1);
z=zeros(length(center(:,1)),1);
if typeNum <10
elseif typeNum <20
    f = rho.*g.*AH(1).*cos(k(1).*center(:,1)-w(1)*t);
    if deepWaterWave == 0
        z=(center(:,3)-elv).*wDepth./(wDepth+elv);
        f = f.*(cosh(k(1).*(z+wDepth))./cosh(k(1)*wDepth));
    else
        z=(center(:,3)-elv);
        f = f.*exp(k(1).*z);
    end
elseif typeNum <30
    for i=1:length(AH)
        if deepWaterWave == 0 && wDepth <= 0.5*pi/k(i)
            z=(center(:,3)-elv).*wDepth./(wDepth+elv);
            f_tmp = rho.*g.*sqrt(AH(i)*dw(i)).*cos(k(i).*center(:,1)-w(i)*t-phaseRand(i));
            f = f + f_tmp.*(cosh(k(i).*(z+wDepth))./cosh(k(i).*wDepth));
        else
            z=(center(:,3)-elv);
            f_tmp = rho.*g.*sqrt(AH(i)*dw(i)).*cos(k(i).*center(:,1)-w(i)*t-phaseRand(i));
            f = f + f_tmp.*exp(k(i).*z);
        end
    end
end
f(z>0)=0;
end

function f = FK(center,instcg,av,wp)
% Function to calculate the force and moment about the cog due to Froude-Krylov pressure
f = zeros(6,1);

% Calculate the hydrostatic pressure at each triangle center
pressureVect = [wp wp wp].*-av;

% Compute force about cog
f(1:3) = sum(pressureVect);

% Compute moment about cog
tmp1 = ones(length(center(:,1)),1);
tmp2 = tmp1*instcg';
center2cgVec = center-tmp2;

f(4:6)= sum(cross(center2cgVec,pressureVect));
end

== matlab function WECSim_Lib/Body Elements/Rigid Body/Non-Hydro Body/Structure/Motion Sensor/Angle ==
  data: Q input; E output
function E  = EulerAngle(Q)
% Euler Angle Type II or Tait-Bryan Angle for sequence 321 or zyx (Nautical or Cardan angles).
% Yaw [-180,180], followed by pitch [-90,90], followed by roll [-180,180]
E = zeros(3,1);
E(1) = atan2( (2*(Q(1)*Q(2)+Q(3)*Q(4))), (1-2* (Q(2)^2+Q(3)^2) ) );
E(2) = asin( 2* (Q(1)*Q(3) - Q(4)*Q(2)));
E(3) = atan2( (2*(Q(1)*Q(4)+Q(2)*Q(3))), (1-2* (Q(3)^2+Q(4)^2) ) );
